simulink model "a_20210406_letturanmea"  (R2020b)
settings: Solver=FixedStepAuto  StartTime=0.0  StopTime=inf  RelTol=1e-3  EnableMultiTasking=on
libraries: arduinolib x1
settings Model: SILPILModeSetting=veronly  ExtModeTrigDuration=2  Creator=ricca  LastModifiedBy=ricca
settings OptimizationCC: EnhancedBackFolding=on  PassReuseOutputArgsAs=Individual arguments  ZeroExternalMemoryAtStartup=off  ZeroInternalMemoryAtStartup=off  MaxStackSize=64  OptimizeBlockOrder=speed  DifferentSizesBufferReuse=on  OptimizationCustomize=off  EfficientTunableParamExpr=on
settings DebuggingCC: ParameterTunabilityLossMsg=error
settings HardwareCC: ProdBitPerPointer=32  ProdBitPerSizeT=32  ProdBitPerPtrDiffT=32  ProdLargestAtomicInteger=Long  ProdLargestAtomicFloat=Double  ProdWordSize=32  ProdHWDeviceType=ARM Compatible->ARM Cortex  UseEmbeddedCoderFeatures=off
settings SFSimCC: MATLABDynamicMemAlloc=off
settings RTWCC: Description=Embedded Coder  SystemTargetFile=ert.tlc  HardwareBoard=Arduino Due  TemplateMakefile=ert_default_tmf  Toolchain=Arduino ARM  BuildConfiguration=Faster Runs
settings CodeAppCC: ForceParamTrailComments=on  IgnoreCustomStorageClasses=off  OperatorAnnotations=on  SimulinkDataObjDesc=on  SFDataObjDesc=on  InsertBlockDesc=on
settings ERTTargetCC: SupportContinuousTime=on  SupportNonInlinedSFcns=on  SupportVariableSizeSignals=on  ExtModeTransport=3  ExtModeStaticAllocSize=24576  ExtModeMexFile=ext_xcp  ExtModeIntrfLevel=Level2 - Open

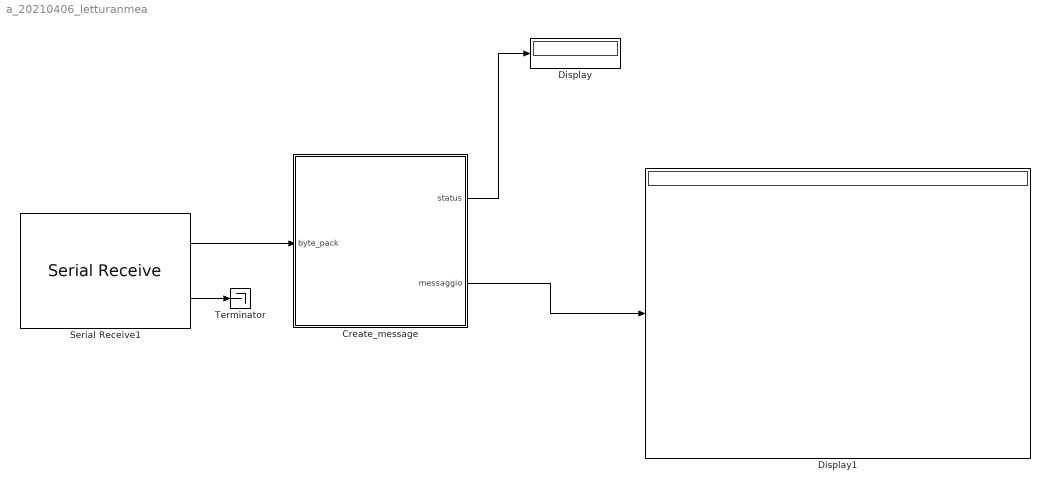
== system a_20210406_letturanmea ==
  Create_message : MATLAB Function  TreatAsAtomicUnit=on
  Display : Display
  Display1 : Display
  Serial Receive1 : arduinolib/Serial Receive  isARMArch=on  portNumber=1  DataType=uint8  Datalength=32  SampleTime=0.02  showOutStatus=on  blockPlatform=arduino
      settings: SourceProductBaseCode=ARDUINO
  Terminator : Terminator
  wires:
  Create_message/1(status) -> Display/1
  Serial Receive1/1 -> Create_message/1(byte_pack)
  Create_message/2(messaggio) -> Display1/1
  Serial Receive1/2 -> Terminator/1

== matlab function a_20210406_letturanmea/Create_message ==
  data: status output; byte_pack input; messaggio output
function [status,messaggio]  = LETTURA_NMEA(byte_pack)

persistent message counter start_found end_found

status = false;       %ho aggiunto questo
messaggio = uint8(zeros(1,80)) ;
pos_end = uint8(0) ;
M = uint8(length(byte_pack)) ;


if isempty(end_found) 
    end_found = false ;
end 
if isempty(start_found) 
     start_found = false ;
end 
if isempty (counter) 
    counter = uint8(0) ;
end 
if isempty(message)
     message = uint8(zeros(1,80)) ;
end



if start_found == 0 
    for i = uint8(1) : M  
        if byte_pack(i) == '$' 
            message(1:M - (i-1)) = byte_pack(i:end) ;
            counter = M - (i-1) ; 
            start_found = true ;
            break
        end
    end
    
    
elseif start_found == 1
    for i = uint8(1) : M  
        if byte_pack(i) == 13 
            end_found = true ;
            pos_end = i ;
            break
        end
    end
    
    if end_found == 1
        message(counter + 1 : counter + pos_end) = byte_pack(1:pos_end) ;
        status = true;       %ho aggiunto questo
        messaggio = message ;
        end_found = false ;
        counter = M - pos_end ;
        if pos_end == M 
            start_found = false ; 
            message = uint8(zeros(1,80)) ;
        else  
            start_found = true ;
            message(1:(M - pos_end)) = byte_pack(pos_end + 1 : end) ;
            message(M - pos_end +1 : 80) = ...
                uint8(zeros(1,80 - (M - pos_end) )) ;
        end
         

    else 
    message(counter + 1 : M + counter ) = byte_pack ;
    counter = M + counter  ;
   
    end
    
    
 
        
    
    
end
